simulink model "BPSK_TX"  (R2018a)
settings: Solver=VariableStepAuto  StartTime=0.0  StopTime=inf  RelTol=1e-3
undefined symbols (not defined in the file): sdrqpsktx
libraries: dspsigops x1, commsequence2 x1, dspsrcs4 x1, commdigbbndpm3 x1, commfilt2 x1, commsdrhw_v2 x1
settings Model: Creator=n53s123  LastModifiedBy=n53s123

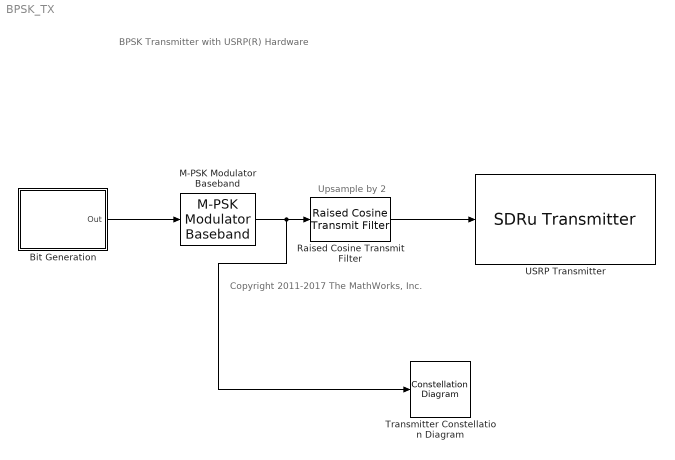
== system BPSK_TX ==
  note: Copyright 2011-2017 The MathWorks, Inc.
  note: BPSK Transmitter with USRP(R) Hardware
  note: Upsample by 2
  Bit Generation : Subsystem
      mask Display: disp('Bits Generation')
  M-PSK Modulator Baseband : commdigbbndpm3/M-PSK Modulator Baseband  M=2  InType=Integer  Enc=Gray  Mapping=[0:7]  Ph=pi  outDtype=double  outWordLen=16  outUDDataType=sfix(16)  outFracLenMode=Best precision  outFracLen=15  outDataTypeStr=double  outLastDataTypeStr=double
      settings: SourceProductName=Communications System Toolbox
  Raised Cosine Transmit Filter : commfilt2/Raised Cosine Transmit Filter  filtType=Square root  R=sdrqpsktx.RolloffFactor  filtSpan=sdrqpsktx.RaisedCosineFilterSpan  N=sdrqpsktx.Interpolation  filterGain=1  InputProcessing=Columns as channels (frame based)  RateOptions=Enforce single-rate processing  framing=Mute  checkCoeff=off  variableName=rcTxFilt1  checkGain=Normalized  sampMode=Mute  saveAsFlag=0  currentFiltSpan=10  D=5  launchFVT=on  roundingMode=Floor  overflowMode=off  coeffDataTypeStr=Inherit: Same word length as input  coeffMin=[]  coeffMax=[]  coeffLastDataTypeStr=Inherit: Same word length as input  outputDataTypeStr=Inherit: Same as accumulator  outputMin=[]  outputMax=[]  outputLastDataTypeStr=Inherit: Same as accumulator
  Transmitter Constellation Diagram : ConstellationDiagram
  USRP Transmitter : commsdrhw_v2/SDRu Transmitter  SourceLibraryInfo="This block requires <a href=\"http://www.mathworks.com/hardware-support/usrp.html\">Communications System Toolbox Support Package for USRP Radio</a>"  rxtx=tx  initializeIPAddress=0  devMap=0  USRP2_IP=192.168.10.2  USRP_IP_X300=192.168.10.2  USRP_IP_X310=192.168.30.2  USRP_serialNumB200=30B2ACA  USRP_serialNumB210=ECR04ZDBT  platform=N200/N210/USRP2  prevPlatform=N200/N210/USRP2  lastIPAddressPopup=192.168.10.2  USRP_ID=192.168.10.2  LastIPAddress=192.168.10.2  ChannelMapping=1  centerFrequencySrc=Dialog  centerFrequency=15000000  loOffsetSrc=Dialog  loOffset=0  gainSrc=Dialog  gain=0  PPSSource=Internal  clockSource=Internal  masterClkRateParam=100e6  masterClkRateB200=sdrqpsktx.MasterClockRate  masterClkRateB210=sdrqpsktx.MasterClockRate  masterClkRateX300=200e6  masterClkRateX310=200e6  decimInterpSrc=Dialog  decimInterp=sdrqpsktx.USRPInterpolationFactor  USRP2_IP_NUM=[49 57 50 46 49 54 56 46 49 48 46 50]  frameLength=362  TransportDataType=int8  outputDatatype=Same as transport data type  overrunUnderrunPort=off  sampleTime=1  dboardInfo=|  HOST_DATA_PORT=30000  HOST_CONTROL_PORT=30001  USRP2_DATA_PORT=32769  USRP2_CONTROL_PORT=32768  bufferMode=Continuous streaming  EnableBurstMode=off  NumFramesInBurst=100
      | dbid: 0
      |           dbName: 'no db found'
      |          freqMin: 0
      |          freqMax: 0
      |          gainMin: 0
      |          gainMax: 0
      |     gainStepSize: 0
      settings: SourceProductName=Communications System Toolbox Support Package for USRP(R) Radio  SourceProductBaseCode=USRP
  wires:
  Raised Cosine Transmit Filter/1 -> USRP Transmitter/1
  M-PSK Modulator Baseband/1 -> Transmitter Constellation Diagram/1, Raised Cosine Transmit Filter/1
  Bit Generation/1(Out) -> M-PSK Modulator Baseband/1

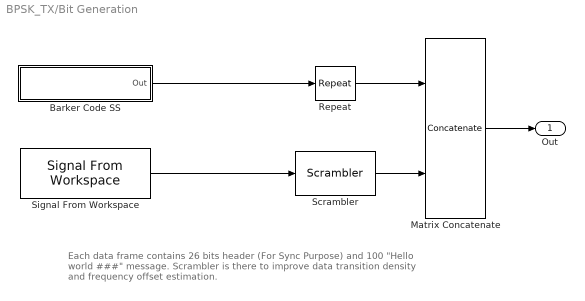
== system BPSK_TX/Bit Generation ==
  note: Each data frame contains 26 bits header (For Sync Purpose) and 100
      | "Hello world ###" message. Scrambler is there to improve data
      | transition density and frequency offset estimation.
  Barker Code SS : Subsystem
      mask Display: disp('Unipolar\nBarker Code')
  Matrix Concatenate : Concatenate  Mode=Multidimensional array
  Repeat : dspsigops/Repeat  N=2  InputProcessing=Columns as channels (frame based)  RateOptions=Enforce single-rate processing  ic=0  mode=Unused parameter value
      settings: SourceProductName=DSP System Toolbox
  Scrambler : commsequence2/Scrambler  M=2  poly=[1 1 1 0 1]  iniStaSource=Dialog Parameter  ini_sta=[0 0 0 0]  resetViaPort=off
      settings: SourceProductName=Communications System Toolbox  SourceProductBaseCode=CM
  Signal From Workspace : dspsrcs4/Signal From Workspace  X=sdrqpsktx.MessageBits  Ts=1/sdrqpsktx.PayloadLength*sdrqpsktx.FrameTime  nsamps=sdrqpsktx.MessageLength * 7 * sdrqpsktx.NumberOfMessage  OutputAfterFinalValue=Cyclic repetition  ignoreOrWarnInputAndFrameLengths=off  OutputFrames=off
  Out : Outport
  wires:
  Barker Code SS/1(Out) -> Repeat/1
  Matrix Concatenate/1 -> Out/1
  Repeat/1 -> Matrix Concatenate/1
  Scrambler/1 -> Matrix Concatenate/2
  Signal From Workspace/1 -> Scrambler/1

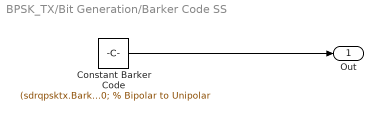
== system BPSK_TX/Bit Generation/Barker Code SS ==
  Constant Barker Code : Constant  Value=(sdrqpsktx.BarkerCode)' > 0; % Bipolar to Unipolar  VectorParams1D=off  OutDataTypeStr=double
  Out : Outport
  wires:
  Constant Barker Code/1 -> Out/1
